simulink model "DIMR_ordinary"  (R2024b)
settings: Solver=daessc  StartTime=0.0  StopTime=20  RelTol=1e-3
values from neighbouring files (symbols this model uses):
  d_m0 = 0.12787808985686    (= 0.127878089857)    [DIMR_main.m]
  d_m_cmd = 0.12787808985686    (= 0.127878089857)    [DIMR_main.m]
  dis_cmd = 3    [DIMR_main.m]
  phi_cmd = 0*pi/180    (= 0)    [DIMR_main.m]
  theta_f0 = 0    [DIMR_main.m]
  theta_f_cmd = 0.037940459    [DIMR_main.m]
  theta_p0 = 0*pi/180    (= 0)    [DIMR_main.m]
  theta_p_cmd = -0.037940459    [DIMR_main.m]
undefined symbols (not defined in the file or in its folder): Ac, Dc, DiscIntNeverNeededParam, dspblkCoreblockFVToolHelper, g, g_ext, g_fork, g_lift, g_reac, g_spado, g_yaw, gcbh, K_fd, K_fp, K_md, K_mp, K_pd, K_pp, K_wd, K_wp, K_yd, K_yp, Kc, L_bx, L_by, L_bz, L_ex, L_ey, L_ez, L_fg, L_fh, L_fx, L_fy, L_fz, L_lx, L_ly, L_lz, L_mx, L_my, L_mz, L_wt, M_f, M_n11, M_n21, M_n22, M_n33, M_n44, Mc, N_f, N_w, omega_c, R_wi, R_wo, T_control, Torque_limit_f, Torque_limit_l, Torque_limit_w, W_w, X, Y ... (+1)
libraries: sm_lib x50, nesl_utility x12, simulink x9, slctrl_autotuning x1, slpidlib x1
(part 3 of 3)

== matlab function DIMR_ordinary/Plant model/MATLAB Function ==
  data: u input; rotx output; roty output; rotz output
function [rotx,roty,rotz] = calculate_rot2eul(u)

rot  = rotm2eul(u);
rotx  = rot(1);
roty  = rot(2);
rotz  = rot(3);

== matlab function DIMR_ordinary/Calc_states/Calc_XY ==
  data: v input; X output; phi input; Xp input; Yp input; Y output
function [X,Y] = fcn(v,phi,Xp,Yp)

X = Xp+v*cos(phi);
Y = Yp+v*sin(phi);

end

== matlab function DIMR_ordinary/Plant model/MBD model/MATLAB Function ==
  data: u input; rotx output; roty output; rotz output
function [rotx,roty,rotz] = calculate_rot2eul(u)

rot  = rotm2eul(u);
rotx  = rot(1);
roty  = rot(2);
rotz  = rot(3);
